simulink model "shadow_test"  (R2023b)
settings: Solver=ode4  StartTime=0.0  StopTime=9  FixedStep=1  RelTol=1e-3
undefined symbols (not defined in the file): AU
libraries: dyn_lib x1
settings Model: Creator=brent  LastModifiedBy=brent

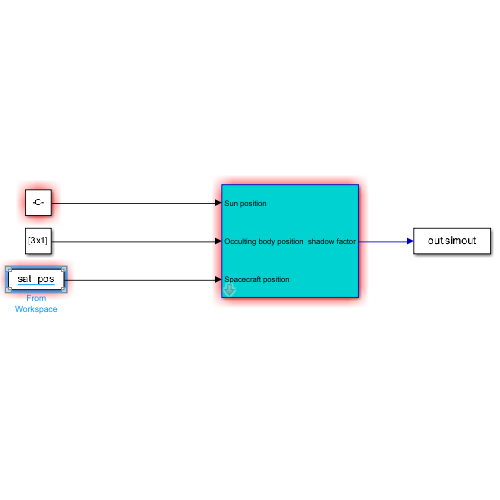
[thumbnail: Simulink's stored preview of the top-level diagram]
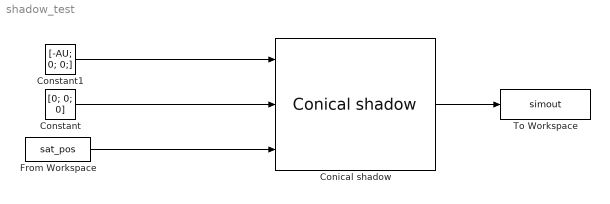
== system shadow_test ==
  Conical shadow : dyn_lib/Conical shadow  R_B=earth_radius  R_S=sun_radius
      settings: SourceProductName=Dynamics library
  Constant : Constant  Value=[0; 0; 0]
  Constant1 : Constant  Value=[-AU; 0; 0;]
  From Workspace : FromWorkspace  VariableName=sat_pos  SampleTime=1
  To Workspace : ToWorkspace  VariableName=simout  SampleTime=-1
      settings: Save2DSignal=2-D array (concatenate along first dimension)
  wires:
  Constant/1 -> Conical shadow/2
  From Workspace/1 -> Conical shadow/3
  Constant1/1 -> Conical shadow/1
  Conical shadow/1 -> To Workspace/1
